simulink model "PID_block"  (R2020b)
settings: Solver=VariableStepAuto  StartTime=0.0  StopTime=120  RelTol=1e-3
model workspace (MAT data in the model file):
  Kd = Simulink.Parameter
  Kd.Value = 10
  Kd.DataType = 'auto'
  Kd.Dimensions = [1 1]
  Ki = Simulink.Parameter
  Ki.Value = 350
  Ki.DataType = 'auto'
  Ki.Dimensions = [1 1]
  Kp = Simulink.Parameter
  Kp.Value = 300
  Kp.DataType = 'auto'
  Kp.Dimensions = [1 1]
settings Model: Creator=Dell  LastModifiedBy=Dell
settings DataIOCC: SaveOutput=off  SaveTime=off

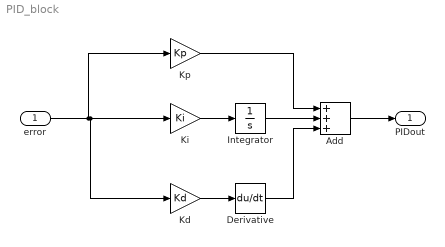
== system PID_block ==
  error : Inport  OutDataTypeStr=double  PortDimensions=1  SampleTime=0
  Add : Sum  Inputs=+++
  Derivative : Derivative
  Integrator : Integrator
  Kd : Gain  Gain=Kd
  Ki : Gain  Gain=Ki
  Kp : Gain  Gain=Kp
  PIDout : Outport  OutDataTypeStr=double  PortDimensions=1  SampleTime=0
  wires:
  error/1 -> Ki/1, Kd/1, Kp/1
  Ki/1 -> Integrator/1
  Integrator/1 -> Add/2
  Kp/1 -> Add/1
  Kd/1 -> Derivative/1
  Derivative/1 -> Add/3
  Add/1 -> PIDout/1
